simulink model "HVPS120_Half_Wave_sfun"  (R2022b)
settings: configuration reference "ModelConfig_var" (kept outside this file)
undefined symbols (not defined in the file or in its folder): InputCircuit
libraries: HVPS_AC120V_HalfWave_sfun_xk x1
settings Model: Creator=KIRTACA  LastModifiedBy=BEDNASA
settings ConfigSetRef: SourceName=ModelConfig_var  SourceLocation=Base Workspace

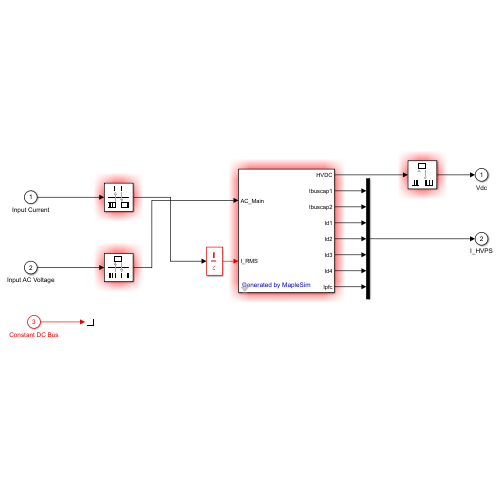
[thumbnail: Simulink's stored preview of the top-level diagram]
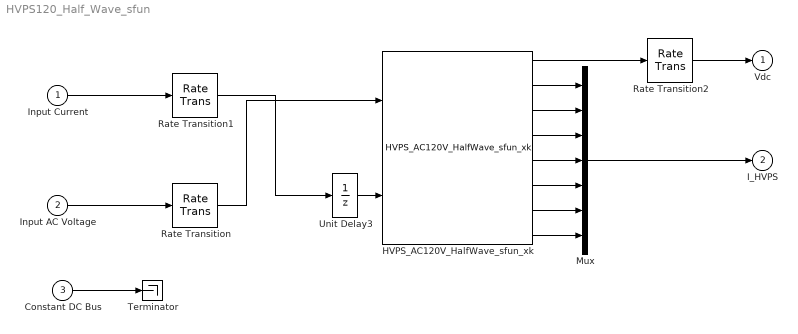
== system HVPS120_Half_Wave_sfun ==
  Input Current : Inport
  Input AC Voltage : Inport  Port=2
  Constant DC Bus : Inport  Port=3
  HVPS_AC120V_HalfWave_sfun_xk : HVPS_AC120V_HalfWave_sfun_xk/HVPS_AC120V_HalfWave_sfun_xk  Description=Subsystem: HVPS_AC120V_HalfWave_sfun_xk  ic=[InputCircuit.Vr*sqrt(2), 0.]  Par1=InputCircuit.C_buscap  Par2=InputCircuit.G_off  Par3=InputCircuit.L_line  Par4=InputCircuit.R_buscap  Par5=InputCircuit.R_diode  Par6=InputCircuit.R_line  Par7=298.15  Par8=0.  Par9=298.15  Par10=0.  Par11=.1e-1  Par12=298.15  Par13=298.15  Par14=.6e6  Par15=298.15  Par16=298.15  Par17=298.15  Par18=298.15  Par19=.4041e-2  Par20=298.15  Par21=298.15  Par22=1.  Par23=1.  Par24=0.  Par25=0.  Par26=.1e4  Par27=TimeSteps.ModelStep  MinStep=1/40  TimeStep_Solver=TimeSteps.ModelStep
  Mux : Mux  Inputs=7
  Rate Transition : RateTransition  InitialCondition=InputCircuit.Vr  OutPortSampleTime=TimeSteps.InputCircuitStep
  Rate Transition1 : RateTransition  OutPortSampleTime=TimeSteps.InputCircuitStep
  Rate Transition2 : RateTransition  InitialCondition=InputCircuit.Vdc_i  OutPortSampleTime=TimeSteps.ModelStep
  Terminator : Terminator
  Unit Delay3 : UnitDelay  SampleTime=-1  HasFrameUpgradeWarning=on
  Vdc : Outport  VectorParamsAs1DForOutWhenUnconnected=off
  I_HVPS : Outport  Port=2  VectorParamsAs1DForOutWhenUnconnected=off
  wires:
  Input AC Voltage/1 -> Rate Transition/1
  Input Current/1 -> Rate Transition1/1
  Rate Transition2/1 -> Vdc/1
  Constant DC Bus/1 -> Terminator/1
  Rate Transition1/1 -> Unit Delay3/1
  Rate Transition/1 -> HVPS_AC120V_HalfWave_sfun_xk/1
  HVPS_AC120V_HalfWave_sfun_xk/1 -> Rate Transition2/1
  Unit Delay3/1 -> HVPS_AC120V_HalfWave_sfun_xk/2
  Mux/1 -> I_HVPS/1
  HVPS_AC120V_HalfWave_sfun_xk/2 -> Mux/1
  HVPS_AC120V_HalfWave_sfun_xk/3 -> Mux/2
  HVPS_AC120V_HalfWave_sfun_xk/4 -> Mux/3
  HVPS_AC120V_HalfWave_sfun_xk/5 -> Mux/4
  HVPS_AC120V_HalfWave_sfun_xk/6 -> Mux/5
  HVPS_AC120V_HalfWave_sfun_xk/7 -> Mux/6
  HVPS_AC120V_HalfWave_sfun_xk/8 -> Mux/7
